simulink model "Ex_Jun_2023"  (R2022b)
settings: Solver=VariableStepAuto  StartTime=0.0  StopTime=200  MaxStep=0.01  RelTol=1e-3
settings Model: Creator=Pablo  LastModifiedBy=rrilo

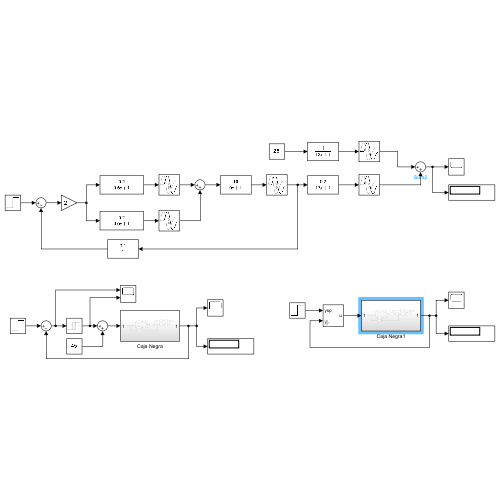
[thumbnail: Simulink's stored preview of the top-level diagram]
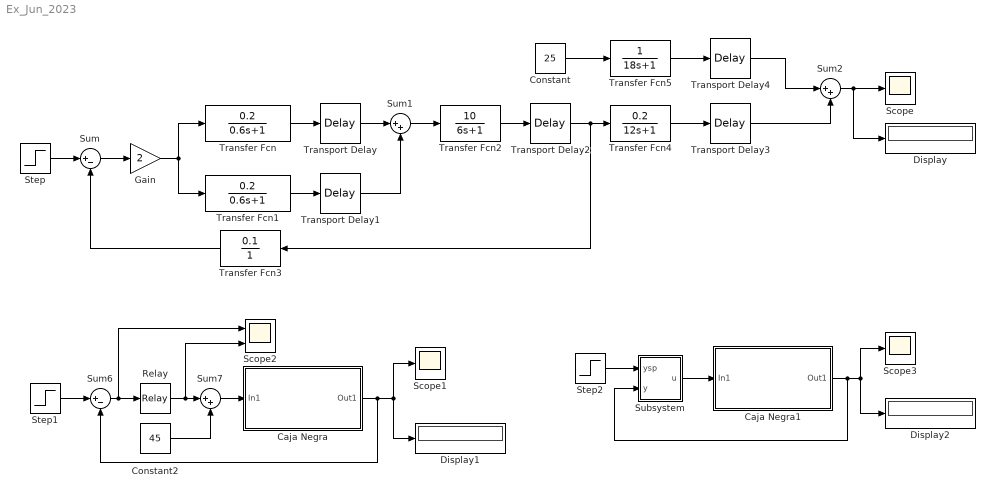
== system Ex_Jun_2023 ==
  Caja Negra : Subsystem
  Caja Negra1 : Subsystem
  Constant : Constant  Value=25
  Constant2 : Constant  Value=45
  Display : Display
  Display1 : Display
  Display2 : Display
  Gain : Gain  Gain=2
  Relay : Relay  OnOutputValue=5  OffOutputValue=-5
  Scope : Scope
  Scope1 : Scope
  Scope2 : Scope  NumInputPorts=2
  Scope3 : Scope
  Step : Step  After=45  SampleTime=0
  Step1 : Step  After=65  SampleTime=0
  Step2 : Step  After=65  SampleTime=0
  Subsystem : Subsystem  mask{Kp=1.908, N=20, Ti=15, Td=3.7375}
  Sum : Sum  Inputs=|+-
  Sum1 : Sum  Inputs=|++
  Sum2 : Sum  Inputs=|++
  Sum6 : Sum  Inputs=|+-
  Sum7 : Sum  Inputs=|++
  Transfer Fcn : TransferFcn  Numerator=[0.2]  Denominator=[0.6 1]
  Transfer Fcn1 : TransferFcn  Numerator=[0.2]  Denominator=[0.6 1]
  Transfer Fcn2 : TransferFcn  Numerator=[10]  Denominator=[6 1]
  Transfer Fcn3 : TransferFcn  Numerator=[0.1]  Denominator=[1]
  Transfer Fcn4 : TransferFcn  Numerator=[0.2]  Denominator=[12 1]
  Transfer Fcn5 : TransferFcn  Denominator=[18 1]
  Transport Delay : TransportDelay  DelayTime=0.2
  Transport Delay1 : TransportDelay  DelayTime=0.5
  Transport Delay2 : TransportDelay
  Transport Delay3 : TransportDelay  DelayTime=5
  Transport Delay4 : TransportDelay  DelayTime=5.5
  wires:
  Sum/1 -> Gain/1
  Gain/1 -> Transfer Fcn/1, Transfer Fcn1/1
  Sum1/1 -> Transfer Fcn2/1
  Transfer Fcn/1 -> Transport Delay/1
  Transport Delay/1 -> Sum1/1
  Transfer Fcn1/1 -> Transport Delay1/1
  Transport Delay1/1 -> Sum1/2
  Transfer Fcn2/1 -> Transport Delay2/1
  Transfer Fcn3/1 -> Sum/2
  Transport Delay2/1 -> Transfer Fcn3/1, Transfer Fcn4/1
  Constant/1 -> Transfer Fcn5/1
  Transfer Fcn5/1 -> Transport Delay4/1
  Step/1 -> Sum/1
  Transport Delay3/1 -> Sum2/2
  Transfer Fcn4/1 -> Transport Delay3/1
  Transport Delay4/1 -> Sum2/1
  Sum2/1 -> Scope/1, Display/1
  Step1/1 -> Sum6/1
  Sum6/1 -> Scope2/1, Relay/1
  Relay/1 -> Scope2/2, Sum7/1
  Constant2/1 -> Sum7/2
  Caja Negra/1(Out1) -> Sum6/2, Display1/1, Scope1/1
  Sum7/1 -> Caja Negra/1(In1)
  Caja Negra1/1(Out1) -> Subsystem/2(y), Display2/1, Scope3/1
  Step2/1 -> Subsystem/1(ysp)
  Subsystem/1(u) -> Caja Negra1/1(In1)

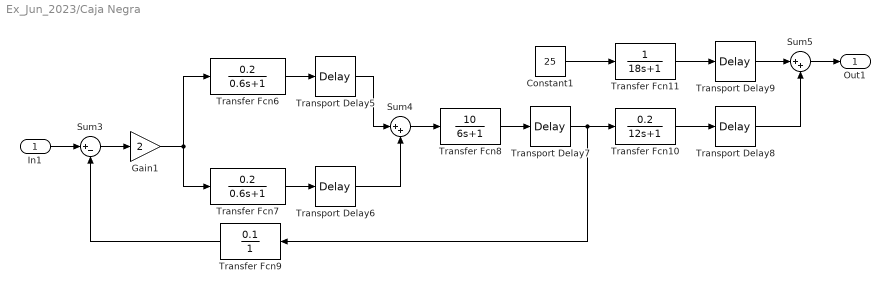
== system Ex_Jun_2023/Caja Negra ==
  In1 : Inport
  Constant1 : Constant  Value=25
  Gain1 : Gain  Gain=2
  Sum3 : Sum  Inputs=|+-
  Sum4 : Sum  Inputs=|++
  Sum5 : Sum  Inputs=|++
  Transfer Fcn10 : TransferFcn  Numerator=[0.2]  Denominator=[12 1]
  Transfer Fcn11 : TransferFcn  Denominator=[18 1]
  Transfer Fcn6 : TransferFcn  Numerator=[0.2]  Denominator=[0.6 1]
  Transfer Fcn7 : TransferFcn  Numerator=[0.2]  Denominator=[0.6 1]
  Transfer Fcn8 : TransferFcn  Numerator=[10]  Denominator=[6 1]
  Transfer Fcn9 : TransferFcn  Numerator=[0.1]  Denominator=[1]
  Transport Delay5 : TransportDelay  DelayTime=0.2
  Transport Delay6 : TransportDelay  DelayTime=0.5
  Transport Delay7 : TransportDelay
  Transport Delay8 : TransportDelay  DelayTime=5
  Transport Delay9 : TransportDelay  DelayTime=5.5
  Out1 : Outport
  wires:
  Transport Delay8/1 -> Sum5/2
  Transfer Fcn11/1 -> Transport Delay9/1
  Gain1/1 -> Transfer Fcn7/1, Transfer Fcn6/1
  Transport Delay7/1 -> Transfer Fcn10/1, Transfer Fcn9/1
  Transport Delay5/1 -> Sum4/1
  Transport Delay9/1 -> Sum5/1
  Sum3/1 -> Gain1/1
  Transfer Fcn10/1 -> Transport Delay8/1
  Transfer Fcn8/1 -> Transport Delay7/1
  Sum5/1 -> Out1/1
  In1/1 -> Sum3/1
  Sum4/1 -> Transfer Fcn8/1
  Constant1/1 -> Transfer Fcn11/1
  Transfer Fcn9/1 -> Sum3/2
  Transport Delay6/1 -> Sum4/2
  Transfer Fcn7/1 -> Transport Delay6/1
  Transfer Fcn6/1 -> Transport Delay5/1

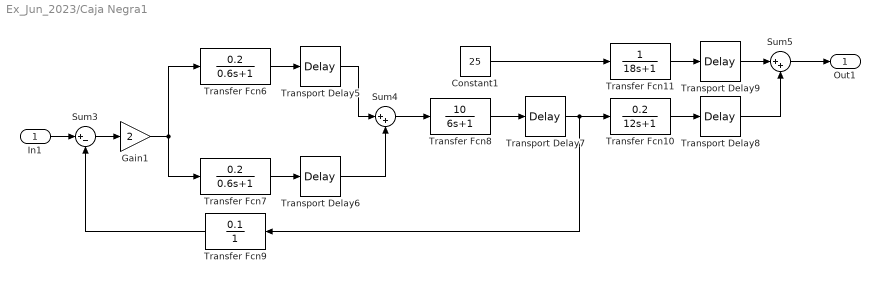
== system Ex_Jun_2023/Caja Negra1 ==
  In1 : Inport
  Constant1 : Constant  Value=25
  Gain1 : Gain  Gain=2
  Sum3 : Sum  Inputs=|+-
  Sum4 : Sum  Inputs=|++
  Sum5 : Sum  Inputs=|++
  Transfer Fcn10 : TransferFcn  Numerator=[0.2]  Denominator=[12 1]
  Transfer Fcn11 : TransferFcn  Denominator=[18 1]
  Transfer Fcn6 : TransferFcn  Numerator=[0.2]  Denominator=[0.6 1]
  Transfer Fcn7 : TransferFcn  Numerator=[0.2]  Denominator=[0.6 1]
  Transfer Fcn8 : TransferFcn  Numerator=[10]  Denominator=[6 1]
  Transfer Fcn9 : TransferFcn  Numerator=[0.1]  Denominator=[1]
  Transport Delay5 : TransportDelay  DelayTime=0.2
  Transport Delay6 : TransportDelay  DelayTime=0.5
  Transport Delay7 : TransportDelay
  Transport Delay8 : TransportDelay  DelayTime=5
  Transport Delay9 : TransportDelay  DelayTime=5.5
  Out1 : Outport
  wires:
  Transport Delay8/1 -> Sum5/2
  Transfer Fcn11/1 -> Transport Delay9/1
  Gain1/1 -> Transfer Fcn7/1, Transfer Fcn6/1
  Transport Delay7/1 -> Transfer Fcn10/1, Transfer Fcn9/1
  Transport Delay5/1 -> Sum4/1
  Transport Delay9/1 -> Sum5/1
  Sum3/1 -> Gain1/1
  Transfer Fcn10/1 -> Transport Delay8/1
  Transfer Fcn8/1 -> Transport Delay7/1
  Sum5/1 -> Out1/1
  In1/1 -> Sum3/1
  Sum4/1 -> Transfer Fcn8/1
  Constant1/1 -> Transfer Fcn11/1
  Transfer Fcn9/1 -> Sum3/2
  Transport Delay6/1 -> Sum4/2
  Transfer Fcn7/1 -> Transport Delay6/1
  Transfer Fcn6/1 -> Transport Delay5/1

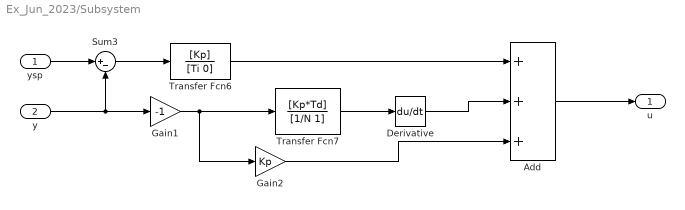
== system Ex_Jun_2023/Subsystem ==
  ysp : Inport
  y : Inport  Port=2
  Add : Sum  Inputs=+++
  Derivative : Derivative
  Gain1 : Gain  Gain=-1
  Gain2 : Gain  Gain=Kp
  Sum3 : Sum  Inputs=|+-
  Transfer Fcn6 : TransferFcn  Numerator=[Kp]  Denominator=[Ti 0]
  Transfer Fcn7 : TransferFcn  Numerator=[Kp*Td]  Denominator=[1/N 1]
  u : Outport
  wires:
  Add/1 -> u/1
  Gain1/1 -> Gain2/1, Transfer Fcn7/1
  Transfer Fcn6/1 -> Add/1
  Sum3/1 -> Transfer Fcn6/1
  Gain2/1 -> Add/3
  Transfer Fcn7/1 -> Derivative/1
  y/1 -> Gain1/1, Sum3/2
  ysp/1 -> Sum3/1
  Derivative/1 -> Add/2
